simulink model "vehicles"  (R2020a)
settings: Solver=VariableStepAuto  StartTime=0.0  StopTime=10.0  RelTol=1e-3
undefined symbols (not defined in the file or in its folder): L, ld, psi_o1, psi_o10, psi_o2, psi_o3, psi_o4, psi_o5, psi_o6, psi_o7, psi_o8, psi_o9, X_last1, X_last10, X_last2, X_last3, X_last4, X_last5, X_last6, X_last7, X_last8, X_last9, X_o, X_o1, X_o10, X_o2, X_o3, X_o4, X_o5, X_o6, X_o7, X_o8, X_o9, xRef1, xRef10, xRef2, xRef3, xRef4, xRef5, xRef6, xRef7, xRef8, xRef9, Y_last1, Y_last10, Y_last2, Y_last3, Y_last4, Y_last5, Y_last6, Y_last7, Y_last8, Y_last9, Y_o, Y_o1, Y_o10, Y_o2, Y_o3, Y_o4, Y_o5 ... (+14)
libraries: autolibutils x40, autolibshared x30, robotalgslib x10, simulink x10, vdynlib x10
(part 1 of 18)
settings Model: Creator=Eskola  LastModifiedBy=Eskola

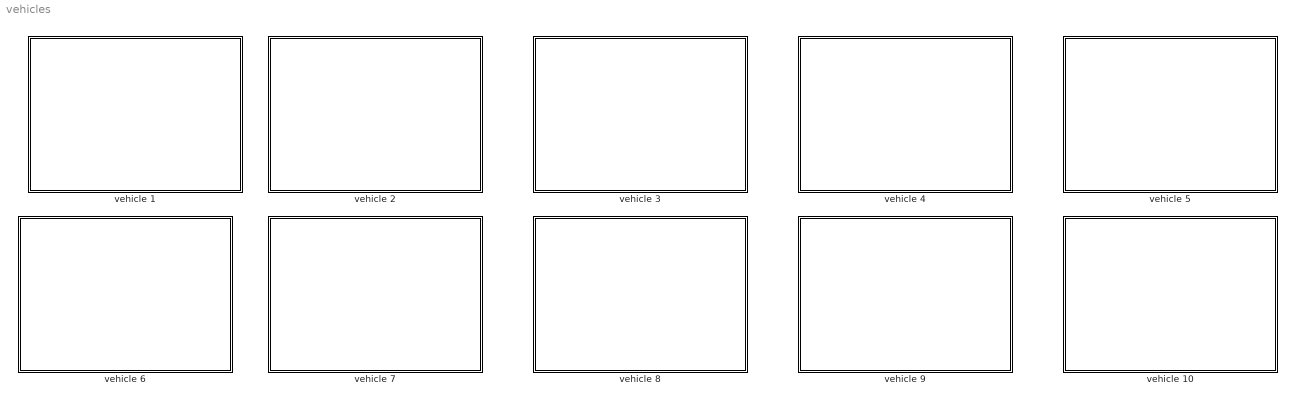
== system vehicles ==
  vehicle 1 : Subsystem
  vehicle 10 : Subsystem
  vehicle 2 : Subsystem
  vehicle 3 : Subsystem
  vehicle 4 : Subsystem
  vehicle 5 : Subsystem
  vehicle 6 : Subsystem
  vehicle 7 : Subsystem
  vehicle 8 : Subsystem
  vehicle 9 : Subsystem

== system vehicles/vehicle 1 ==
  note: Controller
  note: Vehicle Model
  note: Reference
  Bus to Mux1 : Subsystem
  Concatenate1 : Subsystem
  Constant3 : Constant  Value=X_o1
  Constant4 : Constant  Value=Y_o1
  Constant5 : Constant  Value=psi_o1
  Grade1 : Constant  Value=0
  Lateral and Longitudinal Controller1 : Subsystem
  Memory1 : Memory
  Powertrain & Driveline1 : Subsystem
      mask Display: image('vdbslibpt.png');
  Rate Transition1 : Subsystem
  Scope8 : Scope
  Simulation 3D Vehicle with Ground Following1 : vdynlib/Vehicle Scenarios/Sim3D/Sim3D Vehicle/Components/Simulation 3D Vehicle with Ground Following  Priority=-1  PassVehMesh=Small pickup truck  VehColor=Orange  InitialPos=[0,0,0]  InitialRot=[0, 0, 0]  ActorName=SimulinkVehicle1  SampleTime=-1  ActorType=SimulinkVehicle  ID=1  aMode=2  ActorTag=SimulinkVehicle1  CoordinateScheme=SAE
      settings: SourceProductBaseCode=VE
  Terminator{1..3,5..6} (5 alike) : Terminator
  Vehicle Body 3DOF Dual Track1 : autolibshared/Vehicle Body 3DOF Single Track  trackMode=Dual  inputMode=External longitudinal forces  frontSteerMode=on  rearSteerMode=off  windMode=off  muMode=off  extFMode=off  extMMode=off  extXo=on  extpsio=on  extxdoto=off  extro=off  extYo=on  extTamb=off  extydoto=off  aMode=2  NF=2  NR=2  m=2000  a=1.4  b=1.6  h=0.35  X_o=0  xdot_o=0  CalphaMode=off  sigmaMode=on  d=0  w=[1.4,1.4]  Cy_f=12e3  Cy_r=11e3  sigma_f=.1  sigma_r=.1  alpha_f_brk=[-.1 .1]  Cy_f_data=[-9e3 9e3]  alpha_r_brk=[-.1 .1]  Cy_r_data=[-9e3 9e3]  Y_o=0  ydot_o=0  Izz=4000  psi_o=0  r_o=0  Af=2  Cd=.3  Cl=.1  Cpm=.1  beta_w=[0:0.01:0.3]  Cs=[0:0.03:0.9]  Cym=[0:0.01:0.3]  Pabs=101325  Tair=273  g=9.81  mu=1  xdot_tol=.01  Fznom=5000  Fxtire_sat=7e4  Fytire_sat=7e4  longOff=0  latOff=0  vertOff=0  wrapAng=off
      settings: SourceProductBaseCode=PW,MT,VE,VP
  VelRefController1 : Subsystem
  Waypoints1 : Subsystem
  wires:
  Vehicle Body 3DOF Dual Track1/1 -> Rate Transition1/1(Info), Powertrain & Driveline1/3(VehFdbk), Bus to Mux1/1(Info)
  Concatenate1/1(AnF) -> Vehicle Body 3DOF Dual Track1/1
  Bus to Mux1/1(Pose) -> Lateral and Longitudinal Controller1/3(Pose)
  Memory1/1 -> VelRefController1/1(angVel)
  Lateral and Longitudinal Controller1/2(WheelSteeringAngle) -> Concatenate1/1(delta)
  Rate Transition1/3(Yaw) -> Simulation 3D Vehicle with Ground Following1/3
  Lateral and Longitudinal Controller1/4(DecelCmd) -> Powertrain & Driveline1/2(Decel)
  Rate Transition1/2(Y) -> Simulation 3D Vehicle with Ground Following1/2
  Lateral and Longitudinal Controller1/1(angVel) -> Memory1/1
  Bus to Mux1/2(x) -> Lateral and Longitudinal Controller1/6(xCar)
  Lateral and Longitudinal Controller1/3(AcelCmd) -> Powertrain & Driveline1/1(Acc)
  VelRefController1/1(VelRef) -> Lateral and Longitudinal Controller1/4(VelRef)
  Vehicle Body 3DOF Dual Track1/7 -> Terminator6/1
  Vehicle Body 3DOF Dual Track1/3 -> Terminator2/1
  Bus to Mux1/3(y) -> Lateral and Longitudinal Controller1/7(yCar)
  Constant5/1 -> Vehicle Body 3DOF Dual Track1/6
  Vehicle Body 3DOF Dual Track1/6 -> Terminator5/1
  Rate Transition1/1(X) -> Simulation 3D Vehicle with Ground Following1/1
  Powertrain & Driveline1/2(Rear Force) -> Vehicle Body 3DOF Dual Track1/3
  Vehicle Body 3DOF Dual Track1/4 -> Terminator1/1
  Constant3/1 -> Vehicle Body 3DOF Dual Track1/4
  Vehicle Body 3DOF Dual Track1/2 -> Lateral and Longitudinal Controller1/5(VelFdbk), Scope8/1
  Powertrain & Driveline1/1(Front Force) -> Vehicle Body 3DOF Dual Track1/2
  Vehicle Body 3DOF Dual Track1/5 -> Terminator3/1
  Waypoints1/1(WayPoints) -> Lateral and Longitudinal Controller1/1(Waypoints)
  Constant4/1 -> Vehicle Body 3DOF Dual Track1/5
  Grade1/1 -> Lateral and Longitudinal Controller1/2(Grade)

== system vehicles/vehicle 10 ==
  note: Reference
  note: Vehicle Model
  note: Controller
  Bus to Mux1 : Subsystem
  Concatenate1 : Subsystem
  Constant3 : Constant  Value=X_o10
  Constant4 : Constant  Value=Y_o10
  Constant5 : Constant  Value=psi_o10
  Grade1 : Constant  Value=0
  Lateral and Longitudinal Controller1 : Subsystem
  Memory1 : Memory
  Powertrain & Driveline1 : Subsystem
      mask Display: image('vdbslibpt.png');
  Rate Transition1 : Subsystem
  Scope8 : Scope
  Simulation 3D Vehicle with Ground Following1 : vdynlib/Vehicle Scenarios/Sim3D/Sim3D Vehicle/Components/Simulation 3D Vehicle with Ground Following  Priority=-1  PassVehMesh=Box truck  VehColor=Green  InitialPos=[0,0,0]  InitialRot=[0, 0, 0]  ActorName=SimulinkVehicle1  SampleTime=-1  ActorType=SimulinkVehicle  ID=1  aMode=2  ActorTag=SimulinkVehicle1  CoordinateScheme=SAE
      settings: SourceProductBaseCode=VE
  Terminator{1..3,5..6} (5 alike) : Terminator
  Vehicle Body 3DOF Dual Track1 : autolibshared/Vehicle Body 3DOF Single Track  trackMode=Dual  inputMode=External longitudinal forces  frontSteerMode=on  rearSteerMode=off  windMode=off  muMode=off  extFMode=off  extMMode=off  extXo=on  extpsio=on  extxdoto=off  extro=off  extYo=on  extTamb=off  extydoto=off  aMode=2  NF=2  NR=2  m=2000  a=1.4  b=1.6  h=0.35  X_o=0  xdot_o=0  CalphaMode=off  sigmaMode=on  d=0  w=[1.4,1.4]  Cy_f=12e3  Cy_r=11e3  sigma_f=.1  sigma_r=.1  alpha_f_brk=[-.1 .1]  Cy_f_data=[-9e3 9e3]  alpha_r_brk=[-.1 .1]  Cy_r_data=[-9e3 9e3]  Y_o=0  ydot_o=0  Izz=4000  psi_o=0  r_o=0  Af=2  Cd=.3  Cl=.1  Cpm=.1  beta_w=[0:0.01:0.3]  Cs=[0:0.03:0.9]  Cym=[0:0.01:0.3]  Pabs=101325  Tair=273  g=9.81  mu=1  xdot_tol=.01  Fznom=5000  Fxtire_sat=7e4  Fytire_sat=7e4  longOff=0  latOff=0  vertOff=0  wrapAng=off
      settings: SourceProductBaseCode=PW,MT,VE,VP
  VelRefController1 : Subsystem
  Waypoints1 : Subsystem
  wires:
  Grade1/1 -> Lateral and Longitudinal Controller1/2(Grade)
  Constant4/1 -> Vehicle Body 3DOF Dual Track1/5
  Waypoints1/1(WayPoints) -> Lateral and Longitudinal Controller1/1(Waypoints)
  Vehicle Body 3DOF Dual Track1/5 -> Terminator3/1
  Powertrain & Driveline1/1(Front Force) -> Vehicle Body 3DOF Dual Track1/2
  Vehicle Body 3DOF Dual Track1/2 -> Scope8/1, Lateral and Longitudinal Controller1/5(VelFdbk)
  Constant3/1 -> Vehicle Body 3DOF Dual Track1/4
  Vehicle Body 3DOF Dual Track1/4 -> Terminator1/1
  Powertrain & Driveline1/2(Rear Force) -> Vehicle Body 3DOF Dual Track1/3
  Rate Transition1/1(X) -> Simulation 3D Vehicle with Ground Following1/1
  Vehicle Body 3DOF Dual Track1/6 -> Terminator5/1
  Constant5/1 -> Vehicle Body 3DOF Dual Track1/6
  Bus to Mux1/3(y) -> Lateral and Longitudinal Controller1/7(yCar)
  Vehicle Body 3DOF Dual Track1/3 -> Terminator2/1
  Vehicle Body 3DOF Dual Track1/7 -> Terminator6/1
  VelRefController1/1(VelRef) -> Lateral and Longitudinal Controller1/4(VelRef)
  Lateral and Longitudinal Controller1/3(AcelCmd) -> Powertrain & Driveline1/1(Acc)
  Bus to Mux1/2(x) -> Lateral and Longitudinal Controller1/6(xCar)
  Lateral and Longitudinal Controller1/1(angVel) -> Memory1/1
  Rate Transition1/2(Y) -> Simulation 3D Vehicle with Ground Following1/2
  Lateral and Longitudinal Controller1/4(DecelCmd) -> Powertrain & Driveline1/2(Decel)
  Rate Transition1/3(Yaw) -> Simulation 3D Vehicle with Ground Following1/3
  Lateral and Longitudinal Controller1/2(WheelSteeringAngle) -> Concatenate1/1(delta)
  Memory1/1 -> VelRefController1/1(angVel)
  Bus to Mux1/1(Pose) -> Lateral and Longitudinal Controller1/3(Pose)
  Concatenate1/1(AnF) -> Vehicle Body 3DOF Dual Track1/1
  Vehicle Body 3DOF Dual Track1/1 -> Bus to Mux1/1(Info), Powertrain & Driveline1/3(VehFdbk), Rate Transition1/1(Info)

== system vehicles/vehicle 2 ==
  note: Reference
  note: Vehicle Model
  note: Controller
  Bus to Mux1 : Subsystem
  Concatenate1 : Subsystem
  Constant3 : Constant  Value=X_o2
  Constant4 : Constant  Value=Y_o2
  Constant5 : Constant  Value=psi_o2
  Grade1 : Constant  Value=0
  Lateral and Longitudinal Controller1 : Subsystem
  Memory1 : Memory
  Powertrain & Driveline1 : Subsystem
      mask Display: image('vdbslibpt.png');
  Rate Transition1 : Subsystem
  Scope8 : Scope
  Simulation 3D Vehicle with Ground Following1 : vdynlib/Vehicle Scenarios/Sim3D/Sim3D Vehicle/Components/Simulation 3D Vehicle with Ground Following  Priority=-1  PassVehMesh=Muscle car  VehColor=Blue  InitialPos=[0,0,0]  InitialRot=[0, 0, 0]  ActorName=SimulinkVehicle1  SampleTime=-1  ActorType=SimulinkVehicle  ID=1  aMode=2  ActorTag=SimulinkVehicle1  CoordinateScheme=SAE
      settings: SourceProductBaseCode=VE
  Terminator{1..3,5..6} (5 alike) : Terminator
  Vehicle Body 3DOF Dual Track1 : autolibshared/Vehicle Body 3DOF Single Track  trackMode=Dual  inputMode=External longitudinal forces  frontSteerMode=on  rearSteerMode=off  windMode=off  muMode=off  extFMode=off  extMMode=off  extXo=on  extpsio=on  extxdoto=off  extro=off  extYo=on  extTamb=off  extydoto=off  aMode=2  NF=2  NR=2  m=2000  a=1.4  b=1.6  h=0.35  X_o=0  xdot_o=0  CalphaMode=off  sigmaMode=on  d=0  w=[1.4,1.4]  Cy_f=12e3  Cy_r=11e3  sigma_f=.1  sigma_r=.1  alpha_f_brk=[-.1 .1]  Cy_f_data=[-9e3 9e3]  alpha_r_brk=[-.1 .1]  Cy_r_data=[-9e3 9e3]  Y_o=0  ydot_o=0  Izz=4000  psi_o=0  r_o=0  Af=2  Cd=.3  Cl=.1  Cpm=.1  beta_w=[0:0.01:0.3]  Cs=[0:0.03:0.9]  Cym=[0:0.01:0.3]  Pabs=101325  Tair=273  g=9.81  mu=1  xdot_tol=.01  Fznom=5000  Fxtire_sat=7e4  Fytire_sat=7e4  longOff=0  latOff=0  vertOff=0  wrapAng=off
      settings: SourceProductBaseCode=PW,MT,VE,VP
  VelRefController1 : Subsystem
  Waypoints1 : Subsystem
  wires:
  Grade1/1 -> Lateral and Longitudinal Controller1/2(Grade)
  Constant4/1 -> Vehicle Body 3DOF Dual Track1/5
  Waypoints1/1(WayPoints) -> Lateral and Longitudinal Controller1/1(Waypoints)
  Vehicle Body 3DOF Dual Track1/5 -> Terminator3/1
  Powertrain & Driveline1/1(Front Force) -> Vehicle Body 3DOF Dual Track1/2
  Vehicle Body 3DOF Dual Track1/2 -> Scope8/1, Lateral and Longitudinal Controller1/5(VelFdbk)
  Constant3/1 -> Vehicle Body 3DOF Dual Track1/4
  Vehicle Body 3DOF Dual Track1/4 -> Terminator1/1
  Powertrain & Driveline1/2(Rear Force) -> Vehicle Body 3DOF Dual Track1/3
  Rate Transition1/1(X) -> Simulation 3D Vehicle with Ground Following1/1
  Vehicle Body 3DOF Dual Track1/6 -> Terminator5/1
  Constant5/1 -> Vehicle Body 3DOF Dual Track1/6
  Bus to Mux1/3(y) -> Lateral and Longitudinal Controller1/7(yCar)
  Vehicle Body 3DOF Dual Track1/3 -> Terminator2/1
  Vehicle Body 3DOF Dual Track1/7 -> Terminator6/1
  VelRefController1/1(VelRef) -> Lateral and Longitudinal Controller1/4(VelRef)
  Lateral and Longitudinal Controller1/3(AcelCmd) -> Powertrain & Driveline1/1(Acc)
  Bus to Mux1/2(x) -> Lateral and Longitudinal Controller1/6(xCar)
  Lateral and Longitudinal Controller1/1(angVel) -> Memory1/1
  Rate Transition1/2(Y) -> Simulation 3D Vehicle with Ground Following1/2
  Lateral and Longitudinal Controller1/4(DecelCmd) -> Powertrain & Driveline1/2(Decel)
  Rate Transition1/3(Yaw) -> Simulation 3D Vehicle with Ground Following1/3
  Lateral and Longitudinal Controller1/2(WheelSteeringAngle) -> Concatenate1/1(delta)
  Memory1/1 -> VelRefController1/1(angVel)
  Bus to Mux1/1(Pose) -> Lateral and Longitudinal Controller1/3(Pose)
  Concatenate1/1(AnF) -> Vehicle Body 3DOF Dual Track1/1
  Vehicle Body 3DOF Dual Track1/1 -> Bus to Mux1/1(Info), Powertrain & Driveline1/3(VehFdbk), Rate Transition1/1(Info)

== system vehicles/vehicle 3 ==
  note: Controller
  note: Vehicle Model
  note: Reference
  Bus to Mux1 : Subsystem
  Concatenate1 : Subsystem
  Constant3 : Constant  Value=X_o3
  Constant4 : Constant  Value=Y_o3
  Constant5 : Constant  Value=psi_o3
  Grade1 : Constant  Value=0
  Lateral and Longitudinal Controller1 : Subsystem
  Memory1 : Memory
  Powertrain & Driveline1 : Subsystem
      mask Display: image('vdbslibpt.png');
  Rate Transition1 : Subsystem
  Scope8 : Scope
  Simulation 3D Vehicle with Ground Following1 : vdynlib/Vehicle Scenarios/Sim3D/Sim3D Vehicle/Components/Simulation 3D Vehicle with Ground Following  Priority=-1  PassVehMesh=Sedan  VehColor=Black  InitialPos=[0,0,0]  InitialRot=[0, 0, 0]  ActorName=SimulinkVehicle1  SampleTime=-1  ActorType=SimulinkVehicle  ID=1  aMode=2  ActorTag=SimulinkVehicle1  CoordinateScheme=SAE
      settings: SourceProductBaseCode=VE
  Terminator{1..3,5..6} (5 alike) : Terminator
  Vehicle Body 3DOF Dual Track1 : autolibshared/Vehicle Body 3DOF Single Track  trackMode=Dual  inputMode=External longitudinal forces  frontSteerMode=on  rearSteerMode=off  windMode=off  muMode=off  extFMode=off  extMMode=off  extXo=on  extpsio=on  extxdoto=off  extro=off  extYo=on  extTamb=off  extydoto=off  aMode=2  NF=2  NR=2  m=2000  a=1.4  b=1.6  h=0.35  X_o=0  xdot_o=0  CalphaMode=off  sigmaMode=on  d=0  w=[1.4,1.4]  Cy_f=12e3  Cy_r=11e3  sigma_f=.1  sigma_r=.1  alpha_f_brk=[-.1 .1]  Cy_f_data=[-9e3 9e3]  alpha_r_brk=[-.1 .1]  Cy_r_data=[-9e3 9e3]  Y_o=0  ydot_o=0  Izz=4000  psi_o=0  r_o=0  Af=2  Cd=.3  Cl=.1  Cpm=.1  beta_w=[0:0.01:0.3]  Cs=[0:0.03:0.9]  Cym=[0:0.01:0.3]  Pabs=101325  Tair=273  g=9.81  mu=1  xdot_tol=.01  Fznom=5000  Fxtire_sat=7e4  Fytire_sat=7e4  longOff=0  latOff=0  vertOff=0  wrapAng=off
      settings: SourceProductBaseCode=PW,MT,VE,VP
  VelRefController1 : Subsystem
  Waypoints1 : Subsystem
  wires:
  Vehicle Body 3DOF Dual Track1/1 -> Rate Transition1/1(Info), Powertrain & Driveline1/3(VehFdbk), Bus to Mux1/1(Info)
  Concatenate1/1(AnF) -> Vehicle Body 3DOF Dual Track1/1
  Bus to Mux1/1(Pose) -> Lateral and Longitudinal Controller1/3(Pose)
  Memory1/1 -> VelRefController1/1(angVel)
  Lateral and Longitudinal Controller1/2(WheelSteeringAngle) -> Concatenate1/1(delta)
  Rate Transition1/3(Yaw) -> Simulation 3D Vehicle with Ground Following1/3
  Lateral and Longitudinal Controller1/4(DecelCmd) -> Powertrain & Driveline1/2(Decel)
  Rate Transition1/2(Y) -> Simulation 3D Vehicle with Ground Following1/2
  Lateral and Longitudinal Controller1/1(angVel) -> Memory1/1
  Bus to Mux1/2(x) -> Lateral and Longitudinal Controller1/6(xCar)
  Lateral and Longitudinal Controller1/3(AcelCmd) -> Powertrain & Driveline1/1(Acc)
  VelRefController1/1(VelRef) -> Lateral and Longitudinal Controller1/4(VelRef)
  Vehicle Body 3DOF Dual Track1/7 -> Terminator6/1
  Vehicle Body 3DOF Dual Track1/3 -> Terminator2/1
  Bus to Mux1/3(y) -> Lateral and Longitudinal Controller1/7(yCar)
  Constant5/1 -> Vehicle Body 3DOF Dual Track1/6
  Vehicle Body 3DOF Dual Track1/6 -> Terminator5/1
  Rate Transition1/1(X) -> Simulation 3D Vehicle with Ground Following1/1
  Powertrain & Driveline1/2(Rear Force) -> Vehicle Body 3DOF Dual Track1/3
  Vehicle Body 3DOF Dual Track1/4 -> Terminator1/1
  Constant3/1 -> Vehicle Body 3DOF Dual Track1/4
  Vehicle Body 3DOF Dual Track1/2 -> Lateral and Longitudinal Controller1/5(VelFdbk), Scope8/1
  Powertrain & Driveline1/1(Front Force) -> Vehicle Body 3DOF Dual Track1/2
  Vehicle Body 3DOF Dual Track1/5 -> Terminator3/1
  Waypoints1/1(WayPoints) -> Lateral and Longitudinal Controller1/1(Waypoints)
  Constant4/1 -> Vehicle Body 3DOF Dual Track1/5
  Grade1/1 -> Lateral and Longitudinal Controller1/2(Grade)

== system vehicles/vehicle 4 ==
  note: Reference
  note: Vehicle Model
  note: Controller
  Bus to Mux1 : Subsystem
  Concatenate1 : Subsystem
  Constant3 : Constant  Value=X_o4
  Constant4 : Constant  Value=Y_o4
  Constant5 : Constant  Value=psi_o4
  Grade1 : Constant  Value=0
  Lateral and Longitudinal Controller1 : Subsystem
  Memory1 : Memory
  Powertrain & Driveline1 : Subsystem
      mask Display: image('vdbslibpt.png');
  Rate Transition1 : Subsystem
  Scope8 : Scope
  Simulation 3D Vehicle with Ground Following1 : vdynlib/Vehicle Scenarios/Sim3D/Sim3D Vehicle/Components/Simulation 3D Vehicle with Ground Following  Priority=-1  PassVehMesh=Sport utility vehicle  VehColor=Silver  InitialPos=[0,0,0]  InitialRot=[0, 0, 0]  ActorName=SimulinkVehicle2  SampleTime=-1  ActorType=SimulinkVehicle  ID=2  aMode=2  ActorTag=SimulinkVehicle2  CoordinateScheme=SAE
      settings: SourceProductBaseCode=VE
  Terminator{1..3,5..6} (5 alike) : Terminator
  Vehicle Body 3DOF Dual Track1 : autolibshared/Vehicle Body 3DOF Single Track  trackMode=Dual  inputMode=External longitudinal forces  frontSteerMode=on  rearSteerMode=off  windMode=off  muMode=off  extFMode=off  extMMode=off  extXo=on  extpsio=on  extxdoto=off  extro=off  extYo=on  extTamb=off  extydoto=off  aMode=2  NF=2  NR=2  m=2000  a=1.4  b=1.6  h=0.35  X_o=0  xdot_o=0  CalphaMode=off  sigmaMode=on  d=0  w=[1.4,1.4]  Cy_f=12e3  Cy_r=11e3  sigma_f=.1  sigma_r=.1  alpha_f_brk=[-.1 .1]  Cy_f_data=[-9e3 9e3]  alpha_r_brk=[-.1 .1]  Cy_r_data=[-9e3 9e3]  Y_o=0  ydot_o=0  Izz=4000  psi_o=0  r_o=0  Af=2  Cd=.3  Cl=.1  Cpm=.1  beta_w=[0:0.01:0.3]  Cs=[0:0.03:0.9]  Cym=[0:0.01:0.3]  Pabs=101325  Tair=273  g=9.81  mu=1  xdot_tol=.01  Fznom=5000  Fxtire_sat=7e4  Fytire_sat=7e4  longOff=0  latOff=0  vertOff=0  wrapAng=off
      settings: SourceProductBaseCode=PW,MT,VE,VP
  VelRefController1 : Subsystem
  Waypoints1 : Subsystem
  wires:
  Grade1/1 -> Lateral and Longitudinal Controller1/2(Grade)
  Constant4/1 -> Vehicle Body 3DOF Dual Track1/5
  Waypoints1/1(WayPoints) -> Lateral and Longitudinal Controller1/1(Waypoints)
  Vehicle Body 3DOF Dual Track1/5 -> Terminator3/1
  Powertrain & Driveline1/1(Front Force) -> Vehicle Body 3DOF Dual Track1/2
  Vehicle Body 3DOF Dual Track1/2 -> Scope8/1, Lateral and Longitudinal Controller1/5(VelFdbk)
  Constant3/1 -> Vehicle Body 3DOF Dual Track1/4
  Vehicle Body 3DOF Dual Track1/4 -> Terminator1/1
  Powertrain & Driveline1/2(Rear Force) -> Vehicle Body 3DOF Dual Track1/3
  Rate Transition1/1(X) -> Simulation 3D Vehicle with Ground Following1/1
  Vehicle Body 3DOF Dual Track1/6 -> Terminator5/1
  Constant5/1 -> Vehicle Body 3DOF Dual Track1/6
  Bus to Mux1/3(y) -> Lateral and Longitudinal Controller1/7(yCar)
  Vehicle Body 3DOF Dual Track1/3 -> Terminator2/1
  Vehicle Body 3DOF Dual Track1/7 -> Terminator6/1
  VelRefController1/1(VelRef) -> Lateral and Longitudinal Controller1/4(VelRef)
  Lateral and Longitudinal Controller1/3(AcelCmd) -> Powertrain & Driveline1/1(Acc)
  Bus to Mux1/2(x) -> Lateral and Longitudinal Controller1/6(xCar)
  Lateral and Longitudinal Controller1/1(angVel) -> Memory1/1
  Rate Transition1/2(Y) -> Simulation 3D Vehicle with Ground Following1/2
  Lateral and Longitudinal Controller1/4(DecelCmd) -> Powertrain & Driveline1/2(Decel)
  Rate Transition1/3(Yaw) -> Simulation 3D Vehicle with Ground Following1/3
  Lateral and Longitudinal Controller1/2(WheelSteeringAngle) -> Concatenate1/1(delta)
  Memory1/1 -> VelRefController1/1(angVel)
  Bus to Mux1/1(Pose) -> Lateral and Longitudinal Controller1/3(Pose)
  Concatenate1/1(AnF) -> Vehicle Body 3DOF Dual Track1/1
  Vehicle Body 3DOF Dual Track1/1 -> Bus to Mux1/1(Info), Powertrain & Driveline1/3(VehFdbk), Rate Transition1/1(Info)

== system vehicles/vehicle 5 ==
  note: Controller
  note: Vehicle Model
  note: Reference
  Bus to Mux1 : Subsystem
  Concatenate1 : Subsystem
  Constant3 : Constant  Value=X_o5
  Constant4 : Constant  Value=Y_o5
  Constant5 : Constant  Value=psi_o5
  Grade1 : Constant  Value=0
  Lateral and Longitudinal Controller1 : Subsystem
  Memory1 : Memory
  Powertrain & Driveline1 : Subsystem
      mask Display: image('vdbslibpt.png');
  Rate Transition1 : Subsystem
  Scope8 : Scope
  Simulation 3D Vehicle with Ground Following1 : vdynlib/Vehicle Scenarios/Sim3D/Sim3D Vehicle/Components/Simulation 3D Vehicle with Ground Following  Priority=-1  PassVehMesh=Hatchback  VehColor=Red  InitialPos=[0,0,0]  InitialRot=[0, 0, 0]  ActorName=SimulinkVehicle3  SampleTime=-1  ActorType=SimulinkVehicle  ID=3  aMode=2  ActorTag=SimulinkVehicle3  CoordinateScheme=SAE
      settings: SourceProductBaseCode=VE
  Terminator{1..3,5..6} (5 alike) : Terminator
  Vehicle Body 3DOF Dual Track1 : autolibshared/Vehicle Body 3DOF Single Track  trackMode=Dual  inputMode=External longitudinal forces  frontSteerMode=on  rearSteerMode=off  windMode=off  muMode=off  extFMode=off  extMMode=off  extXo=on  extpsio=on  extxdoto=off  extro=off  extYo=on  extTamb=off  extydoto=off  aMode=2  NF=2  NR=2  m=2000  a=1.4  b=1.6  h=0.35  X_o=0  xdot_o=0  CalphaMode=off  sigmaMode=on  d=0  w=[1.4,1.4]  Cy_f=12e3  Cy_r=11e3  sigma_f=.1  sigma_r=.1  alpha_f_brk=[-.1 .1]  Cy_f_data=[-9e3 9e3]  alpha_r_brk=[-.1 .1]  Cy_r_data=[-9e3 9e3]  Y_o=0  ydot_o=0  Izz=4000  psi_o=0  r_o=0  Af=2  Cd=.3  Cl=.1  Cpm=.1  beta_w=[0:0.01:0.3]  Cs=[0:0.03:0.9]  Cym=[0:0.01:0.3]  Pabs=101325  Tair=273  g=9.81  mu=1  xdot_tol=.01  Fznom=5000  Fxtire_sat=7e4  Fytire_sat=7e4  longOff=0  latOff=0  vertOff=0  wrapAng=off
      settings: SourceProductBaseCode=PW,MT,VE,VP
  VelRefController1 : Subsystem
  Waypoints1 : Subsystem
  wires:
  Vehicle Body 3DOF Dual Track1/1 -> Rate Transition1/1(Info), Powertrain & Driveline1/3(VehFdbk), Bus to Mux1/1(Info)
  Concatenate1/1(AnF) -> Vehicle Body 3DOF Dual Track1/1
  Bus to Mux1/1(Pose) -> Lateral and Longitudinal Controller1/3(Pose)
  Memory1/1 -> VelRefController1/1(angVel)
  Lateral and Longitudinal Controller1/2(WheelSteeringAngle) -> Concatenate1/1(delta)
  Rate Transition1/3(Yaw) -> Simulation 3D Vehicle with Ground Following1/3
  Lateral and Longitudinal Controller1/4(DecelCmd) -> Powertrain & Driveline1/2(Decel)
  Rate Transition1/2(Y) -> Simulation 3D Vehicle with Ground Following1/2
  Lateral and Longitudinal Controller1/1(angVel) -> Memory1/1
  Bus to Mux1/2(x) -> Lateral and Longitudinal Controller1/6(xCar)
  Lateral and Longitudinal Controller1/3(AcelCmd) -> Powertrain & Driveline1/1(Acc)
  VelRefController1/1(VelRef) -> Lateral and Longitudinal Controller1/4(VelRef)
  Vehicle Body 3DOF Dual Track1/7 -> Terminator6/1
  Vehicle Body 3DOF Dual Track1/3 -> Terminator2/1
  Bus to Mux1/3(y) -> Lateral and Longitudinal Controller1/7(yCar)
  Constant5/1 -> Vehicle Body 3DOF Dual Track1/6
  Vehicle Body 3DOF Dual Track1/6 -> Terminator5/1
  Rate Transition1/1(X) -> Simulation 3D Vehicle with Ground Following1/1
  Powertrain & Driveline1/2(Rear Force) -> Vehicle Body 3DOF Dual Track1/3
  Vehicle Body 3DOF Dual Track1/4 -> Terminator1/1
  Constant3/1 -> Vehicle Body 3DOF Dual Track1/4
  Vehicle Body 3DOF Dual Track1/2 -> Lateral and Longitudinal Controller1/5(VelFdbk), Scope8/1
  Powertrain & Driveline1/1(Front Force) -> Vehicle Body 3DOF Dual Track1/2
  Vehicle Body 3DOF Dual Track1/5 -> Terminator3/1
  Waypoints1/1(WayPoints) -> Lateral and Longitudinal Controller1/1(Waypoints)
  Constant4/1 -> Vehicle Body 3DOF Dual Track1/5
  Grade1/1 -> Lateral and Longitudinal Controller1/2(Grade)

== system vehicles/vehicle 6 ==
  note: Reference
  note: Vehicle Model
  note: Controller
  Bus to Mux1 : Subsystem
  Concatenate1 : Subsystem
  Constant3 : Constant  Value=X_o6
  Constant4 : Constant  Value=Y_o6
  Constant5 : Constant  Value=psi_o6
  Grade1 : Constant  Value=0
  Lateral and Longitudinal Controller1 : Subsystem
  Memory1 : Memory
  Powertrain & Driveline1 : Subsystem
      mask Display: image('vdbslibpt.png');
  Rate Transition1 : Subsystem
  Scope8 : Scope
  Simulation 3D Vehicle with Ground Following1 : vdynlib/Vehicle Scenarios/Sim3D/Sim3D Vehicle/Components/Simulation 3D Vehicle with Ground Following  Priority=-1  PassVehMesh=Box truck  VehColor=Green  InitialPos=[0,0,0]  InitialRot=[0, 0, 0]  ActorName=SimulinkVehicle2  SampleTime=-1  ActorType=SimulinkVehicle  ID=2  aMode=2  ActorTag=SimulinkVehicle2  CoordinateScheme=SAE
      settings: SourceProductBaseCode=VE
  Terminator{1..3,5..6} (5 alike) : Terminator
  Vehicle Body 3DOF Dual Track1 : autolibshared/Vehicle Body 3DOF Single Track  trackMode=Dual  inputMode=External longitudinal forces  frontSteerMode=on  rearSteerMode=off  windMode=off  muMode=off  extFMode=off  extMMode=off  extXo=on  extpsio=on  extxdoto=off  extro=off  extYo=on  extTamb=off  extydoto=off  aMode=2  NF=2  NR=2  m=2000  a=1.4  b=1.6  h=0.35  X_o=0  xdot_o=0  CalphaMode=off  sigmaMode=on  d=0  w=[1.4,1.4]  Cy_f=12e3  Cy_r=11e3  sigma_f=.1  sigma_r=.1  alpha_f_brk=[-.1 .1]  Cy_f_data=[-9e3 9e3]  alpha_r_brk=[-.1 .1]  Cy_r_data=[-9e3 9e3]  Y_o=0  ydot_o=0  Izz=4000  psi_o=0  r_o=0  Af=2  Cd=.3  Cl=.1  Cpm=.1  beta_w=[0:0.01:0.3]  Cs=[0:0.03:0.9]  Cym=[0:0.01:0.3]  Pabs=101325  Tair=273  g=9.81  mu=1  xdot_tol=.01  Fznom=5000  Fxtire_sat=7e4  Fytire_sat=7e4  longOff=0  latOff=0  vertOff=0  wrapAng=off
      settings: SourceProductBaseCode=PW,MT,VE,VP
  VelRefController1 : Subsystem
  Waypoints1 : Subsystem
  wires:
  Grade1/1 -> Lateral and Longitudinal Controller1/2(Grade)
  Constant4/1 -> Vehicle Body 3DOF Dual Track1/5
  Waypoints1/1(WayPoints) -> Lateral and Longitudinal Controller1/1(Waypoints)
  Vehicle Body 3DOF Dual Track1/5 -> Terminator3/1
  Powertrain & Driveline1/1(Front Force) -> Vehicle Body 3DOF Dual Track1/2
  Vehicle Body 3DOF Dual Track1/2 -> Scope8/1, Lateral and Longitudinal Controller1/5(VelFdbk)
  Constant3/1 -> Vehicle Body 3DOF Dual Track1/4
  Vehicle Body 3DOF Dual Track1/4 -> Terminator1/1
  Powertrain & Driveline1/2(Rear Force) -> Vehicle Body 3DOF Dual Track1/3
  Rate Transition1/1(X) -> Simulation 3D Vehicle with Ground Following1/1
  Vehicle Body 3DOF Dual Track1/6 -> Terminator5/1
  Constant5/1 -> Vehicle Body 3DOF Dual Track1/6
  Bus to Mux1/3(y) -> Lateral and Longitudinal Controller1/7(yCar)
  Vehicle Body 3DOF Dual Track1/3 -> Terminator2/1
  Vehicle Body 3DOF Dual Track1/7 -> Terminator6/1
  VelRefController1/1(VelRef) -> Lateral and Longitudinal Controller1/4(VelRef)
  Lateral and Longitudinal Controller1/3(AcelCmd) -> Powertrain & Driveline1/1(Acc)
  Bus to Mux1/2(x) -> Lateral and Longitudinal Controller1/6(xCar)
  Lateral and Longitudinal Controller1/1(angVel) -> Memory1/1
  Rate Transition1/2(Y) -> Simulation 3D Vehicle with Ground Following1/2
  Lateral and Longitudinal Controller1/4(DecelCmd) -> Powertrain & Driveline1/2(Decel)
  Rate Transition1/3(Yaw) -> Simulation 3D Vehicle with Ground Following1/3
  Lateral and Longitudinal Controller1/2(WheelSteeringAngle) -> Concatenate1/1(delta)
  Memory1/1 -> VelRefController1/1(angVel)
  Bus to Mux1/1(Pose) -> Lateral and Longitudinal Controller1/3(Pose)
  Concatenate1/1(AnF) -> Vehicle Body 3DOF Dual Track1/1
  Vehicle Body 3DOF Dual Track1/1 -> Bus to Mux1/1(Info), Powertrain & Driveline1/3(VehFdbk), Rate Transition1/1(Info)

== system vehicles/vehicle 7 ==
  note: Controller
  note: Vehicle Model
  note: Reference
  Bus to Mux1 : Subsystem
  Concatenate1 : Subsystem
  Constant3 : Constant  Value=X_o7
  Constant4 : Constant  Value=Y_o7
  Constant5 : Constant  Value=psi_o7
  Grade1 : Constant  Value=0
  Lateral and Longitudinal Controller1 : Subsystem
  Memory1 : Memory
  Powertrain & Driveline1 : Subsystem
      mask Display: image('vdbslibpt.png');
  Rate Transition1 : Subsystem
  Scope8 : Scope
  Simulation 3D Vehicle with Ground Following1 : vdynlib/Vehicle Scenarios/Sim3D/Sim3D Vehicle/Components/Simulation 3D Vehicle with Ground Following  Priority=-1  PassVehMesh=Box truck  VehColor=Green  InitialPos=[0,0,0]  InitialRot=[0, 0, 0]  ActorName=SimulinkVehicle3  SampleTime=-1  ActorType=SimulinkVehicle  ID=3  aMode=2  ActorTag=SimulinkVehicle3  CoordinateScheme=SAE
      settings: SourceProductBaseCode=VE
  Terminator{1..3,5..6} (5 alike) : Terminator
  Vehicle Body 3DOF Dual Track1 : autolibshared/Vehicle Body 3DOF Single Track  trackMode=Dual  inputMode=External longitudinal forces  frontSteerMode=on  rearSteerMode=off  windMode=off  muMode=off  extFMode=off  extMMode=off  extXo=on  extpsio=on  extxdoto=off  extro=off  extYo=on  extTamb=off  extydoto=off  aMode=2  NF=2  NR=2  m=2000  a=1.4  b=1.6  h=0.35  X_o=0  xdot_o=0  CalphaMode=off  sigmaMode=on  d=0  w=[1.4,1.4]  Cy_f=12e3  Cy_r=11e3  sigma_f=.1  sigma_r=.1  alpha_f_brk=[-.1 .1]  Cy_f_data=[-9e3 9e3]  alpha_r_brk=[-.1 .1]  Cy_r_data=[-9e3 9e3]  Y_o=0  ydot_o=0  Izz=4000  psi_o=0  r_o=0  Af=2  Cd=.3  Cl=.1  Cpm=.1  beta_w=[0:0.01:0.3]  Cs=[0:0.03:0.9]  Cym=[0:0.01:0.3]  Pabs=101325  Tair=273  g=9.81  mu=1  xdot_tol=.01  Fznom=5000  Fxtire_sat=7e4  Fytire_sat=7e4  longOff=0  latOff=0  vertOff=0  wrapAng=off
      settings: SourceProductBaseCode=PW,MT,VE,VP
  VelRefController1 : Subsystem
  Waypoints1 : Subsystem
  wires:
  Vehicle Body 3DOF Dual Track1/1 -> Rate Transition1/1(Info), Powertrain & Driveline1/3(VehFdbk), Bus to Mux1/1(Info)
  Concatenate1/1(AnF) -> Vehicle Body 3DOF Dual Track1/1
  Bus to Mux1/1(Pose) -> Lateral and Longitudinal Controller1/3(Pose)
  Memory1/1 -> VelRefController1/1(angVel)
  Lateral and Longitudinal Controller1/2(WheelSteeringAngle) -> Concatenate1/1(delta)
  Rate Transition1/3(Yaw) -> Simulation 3D Vehicle with Ground Following1/3
  Lateral and Longitudinal Controller1/4(DecelCmd) -> Powertrain & Driveline1/2(Decel)
  Rate Transition1/2(Y) -> Simulation 3D Vehicle with Ground Following1/2
  Lateral and Longitudinal Controller1/1(angVel) -> Memory1/1
  Bus to Mux1/2(x) -> Lateral and Longitudinal Controller1/6(xCar)
  Lateral and Longitudinal Controller1/3(AcelCmd) -> Powertrain & Driveline1/1(Acc)
  VelRefController1/1(VelRef) -> Lateral and Longitudinal Controller1/4(VelRef)
  Vehicle Body 3DOF Dual Track1/7 -> Terminator6/1
  Vehicle Body 3DOF Dual Track1/3 -> Terminator2/1
  Bus to Mux1/3(y) -> Lateral and Longitudinal Controller1/7(yCar)
  Constant5/1 -> Vehicle Body 3DOF Dual Track1/6
  Vehicle Body 3DOF Dual Track1/6 -> Terminator5/1
  Rate Transition1/1(X) -> Simulation 3D Vehicle with Ground Following1/1
  Powertrain & Driveline1/2(Rear Force) -> Vehicle Body 3DOF Dual Track1/3
  Vehicle Body 3DOF Dual Track1/4 -> Terminator1/1
  Constant3/1 -> Vehicle Body 3DOF Dual Track1/4
  Vehicle Body 3DOF Dual Track1/2 -> Lateral and Longitudinal Controller1/5(VelFdbk), Scope8/1
  Powertrain & Driveline1/1(Front Force) -> Vehicle Body 3DOF Dual Track1/2
  Vehicle Body 3DOF Dual Track1/5 -> Terminator3/1
  Waypoints1/1(WayPoints) -> Lateral and Longitudinal Controller1/1(Waypoints)
  Constant4/1 -> Vehicle Body 3DOF Dual Track1/5
  Grade1/1 -> Lateral and Longitudinal Controller1/2(Grade)

== system vehicles/vehicle 8 ==
  note: Reference
  note: Vehicle Model
  note: Controller
  Bus to Mux1 : Subsystem
  Concatenate1 : Subsystem
  Constant3 : Constant  Value=X_o8
  Constant4 : Constant  Value=Y_o8
  Constant5 : Constant  Value=psi_o8
  Grade1 : Constant  Value=0
  Lateral and Longitudinal Controller1 : Subsystem
  Memory1 : Memory
  Powertrain & Driveline1 : Subsystem
      mask Display: image('vdbslibpt.png');
  Rate Transition1 : Subsystem
  Scope8 : Scope
  Simulation 3D Vehicle with Ground Following1 : vdynlib/Vehicle Scenarios/Sim3D/Sim3D Vehicle/Components/Simulation 3D Vehicle with Ground Following  Priority=-1  PassVehMesh=Box truck  VehColor=Green  InitialPos=[0,0,0]  InitialRot=[0, 0, 0]  ActorName=SimulinkVehicle4  SampleTime=-1  ActorType=SimulinkVehicle  ID=4  aMode=2  ActorTag=SimulinkVehicle4  CoordinateScheme=SAE
      settings: SourceProductBaseCode=VE
  Terminator{1..3,5..6} (5 alike) : Terminator
  Vehicle Body 3DOF Dual Track1 : autolibshared/Vehicle Body 3DOF Single Track  trackMode=Dual  inputMode=External longitudinal forces  frontSteerMode=on  rearSteerMode=off  windMode=off  muMode=off  extFMode=off  extMMode=off  extXo=on  extpsio=on  extxdoto=off  extro=off  extYo=on  extTamb=off  extydoto=off  aMode=2  NF=2  NR=2  m=2000  a=1.4  b=1.6  h=0.35  X_o=0  xdot_o=0  CalphaMode=off  sigmaMode=on  d=0  w=[1.4,1.4]  Cy_f=12e3  Cy_r=11e3  sigma_f=.1  sigma_r=.1  alpha_f_brk=[-.1 .1]  Cy_f_data=[-9e3 9e3]  alpha_r_brk=[-.1 .1]  Cy_r_data=[-9e3 9e3]  Y_o=0  ydot_o=0  Izz=4000  psi_o=0  r_o=0  Af=2  Cd=.3  Cl=.1  Cpm=.1  beta_w=[0:0.01:0.3]  Cs=[0:0.03:0.9]  Cym=[0:0.01:0.3]  Pabs=101325  Tair=273  g=9.81  mu=1  xdot_tol=.01  Fznom=5000  Fxtire_sat=7e4  Fytire_sat=7e4  longOff=0  latOff=0  vertOff=0  wrapAng=off
      settings: SourceProductBaseCode=PW,MT,VE,VP
  VelRefController1 : Subsystem
  Waypoints1 : Subsystem
  wires:
  Grade1/1 -> Lateral and Longitudinal Controller1/2(Grade)
  Constant4/1 -> Vehicle Body 3DOF Dual Track1/5
  Waypoints1/1(WayPoints) -> Lateral and Longitudinal Controller1/1(Waypoints)
  Vehicle Body 3DOF Dual Track1/5 -> Terminator3/1
  Powertrain & Driveline1/1(Front Force) -> Vehicle Body 3DOF Dual Track1/2
  Vehicle Body 3DOF Dual Track1/2 -> Scope8/1, Lateral and Longitudinal Controller1/5(VelFdbk)
  Constant3/1 -> Vehicle Body 3DOF Dual Track1/4
  Vehicle Body 3DOF Dual Track1/4 -> Terminator1/1
  Powertrain & Driveline1/2(Rear Force) -> Vehicle Body 3DOF Dual Track1/3
  Rate Transition1/1(X) -> Simulation 3D Vehicle with Ground Following1/1
  Vehicle Body 3DOF Dual Track1/6 -> Terminator5/1
  Constant5/1 -> Vehicle Body 3DOF Dual Track1/6
  Bus to Mux1/3(y) -> Lateral and Longitudinal Controller1/7(yCar)
  Vehicle Body 3DOF Dual Track1/3 -> Terminator2/1
  Vehicle Body 3DOF Dual Track1/7 -> Terminator6/1
  VelRefController1/1(VelRef) -> Lateral and Longitudinal Controller1/4(VelRef)
  Lateral and Longitudinal Controller1/3(AcelCmd) -> Powertrain & Driveline1/1(Acc)
  Bus to Mux1/2(x) -> Lateral and Longitudinal Controller1/6(xCar)
  Lateral and Longitudinal Controller1/1(angVel) -> Memory1/1
  Rate Transition1/2(Y) -> Simulation 3D Vehicle with Ground Following1/2
  Lateral and Longitudinal Controller1/4(DecelCmd) -> Powertrain & Driveline1/2(Decel)
  Rate Transition1/3(Yaw) -> Simulation 3D Vehicle with Ground Following1/3
  Lateral and Longitudinal Controller1/2(WheelSteeringAngle) -> Concatenate1/1(delta)
  Memory1/1 -> VelRefController1/1(angVel)
  Bus to Mux1/1(Pose) -> Lateral and Longitudinal Controller1/3(Pose)
  Concatenate1/1(AnF) -> Vehicle Body 3DOF Dual Track1/1
  Vehicle Body 3DOF Dual Track1/1 -> Bus to Mux1/1(Info), Powertrain & Driveline1/3(VehFdbk), Rate Transition1/1(Info)

== system vehicles/vehicle 9 ==
  note: Controller
  note: Vehicle Model
  note: Reference
  Bus to Mux1 : Subsystem
  Concatenate1 : Subsystem
  Constant3 : Constant  Value=X_o9
  Constant4 : Constant  Value=Y_o9
  Constant5 : Constant  Value=psi_o9
  Grade1 : Constant  Value=0
  Lateral and Longitudinal Controller1 : Subsystem
  Memory1 : Memory
  Powertrain & Driveline1 : Subsystem
      mask Display: image('vdbslibpt.png');
  Rate Transition1 : Subsystem
  Scope8 : Scope
  Simulation 3D Vehicle with Ground Following1 : vdynlib/Vehicle Scenarios/Sim3D/Sim3D Vehicle/Components/Simulation 3D Vehicle with Ground Following  Priority=-1  PassVehMesh=Box truck  VehColor=Green  InitialPos=[0,0,0]  InitialRot=[0, 0, 0]  ActorName=SimulinkVehicle5  SampleTime=-1  ActorType=SimulinkVehicle  ID=5  aMode=2  ActorTag=SimulinkVehicle5  CoordinateScheme=SAE
      settings: SourceProductBaseCode=VE
  Terminator{1..3,5..6} (5 alike) : Terminator
  Vehicle Body 3DOF Dual Track1 : autolibshared/Vehicle Body 3DOF Single Track  trackMode=Dual  inputMode=External longitudinal forces  frontSteerMode=on  rearSteerMode=off  windMode=off  muMode=off  extFMode=off  extMMode=off  extXo=on  extpsio=on  extxdoto=off  extro=off  extYo=on  extTamb=off  extydoto=off  aMode=2  NF=2  NR=2  m=2000  a=1.4  b=1.6  h=0.35  X_o=0  xdot_o=0  CalphaMode=off  sigmaMode=on  d=0  w=[1.4,1.4]  Cy_f=12e3  Cy_r=11e3  sigma_f=.1  sigma_r=.1  alpha_f_brk=[-.1 .1]  Cy_f_data=[-9e3 9e3]  alpha_r_brk=[-.1 .1]  Cy_r_data=[-9e3 9e3]  Y_o=0  ydot_o=0  Izz=4000  psi_o=0  r_o=0  Af=2  Cd=.3  Cl=.1  Cpm=.1  beta_w=[0:0.01:0.3]  Cs=[0:0.03:0.9]  Cym=[0:0.01:0.3]  Pabs=101325  Tair=273  g=9.81  mu=1  xdot_tol=.01  Fznom=5000  Fxtire_sat=7e4  Fytire_sat=7e4  longOff=0  latOff=0  vertOff=0  wrapAng=off
      settings: SourceProductBaseCode=PW,MT,VE,VP
  VelRefController1 : Subsystem
  Waypoints1 : Subsystem
  wires:
  Vehicle Body 3DOF Dual Track1/1 -> Rate Transition1/1(Info), Powertrain & Driveline1/3(VehFdbk), Bus to Mux1/1(Info)
  Concatenate1/1(AnF) -> Vehicle Body 3DOF Dual Track1/1
  Bus to Mux1/1(Pose) -> Lateral and Longitudinal Controller1/3(Pose)
  Memory1/1 -> VelRefController1/1(angVel)
  Lateral and Longitudinal Controller1/2(WheelSteeringAngle) -> Concatenate1/1(delta)
  Rate Transition1/3(Yaw) -> Simulation 3D Vehicle with Ground Following1/3
  Lateral and Longitudinal Controller1/4(DecelCmd) -> Powertrain & Driveline1/2(Decel)
  Rate Transition1/2(Y) -> Simulation 3D Vehicle with Ground Following1/2
  Lateral and Longitudinal Controller1/1(angVel) -> Memory1/1
  Bus to Mux1/2(x) -> Lateral and Longitudinal Controller1/6(xCar)
  Lateral and Longitudinal Controller1/3(AcelCmd) -> Powertrain & Driveline1/1(Acc)
  VelRefController1/1(VelRef) -> Lateral and Longitudinal Controller1/4(VelRef)
  Vehicle Body 3DOF Dual Track1/7 -> Terminator6/1
  Vehicle Body 3DOF Dual Track1/3 -> Terminator2/1
  Bus to Mux1/3(y) -> Lateral and Longitudinal Controller1/7(yCar)
  Constant5/1 -> Vehicle Body 3DOF Dual Track1/6
  Vehicle Body 3DOF Dual Track1/6 -> Terminator5/1
  Rate Transition1/1(X) -> Simulation 3D Vehicle with Ground Following1/1
  Powertrain & Driveline1/2(Rear Force) -> Vehicle Body 3DOF Dual Track1/3
  Vehicle Body 3DOF Dual Track1/4 -> Terminator1/1
  Constant3/1 -> Vehicle Body 3DOF Dual Track1/4
  Vehicle Body 3DOF Dual Track1/2 -> Lateral and Longitudinal Controller1/5(VelFdbk), Scope8/1
  Powertrain & Driveline1/1(Front Force) -> Vehicle Body 3DOF Dual Track1/2
  Vehicle Body 3DOF Dual Track1/5 -> Terminator3/1
  Waypoints1/1(WayPoints) -> Lateral and Longitudinal Controller1/1(Waypoints)
  Constant4/1 -> Vehicle Body 3DOF Dual Track1/5
  Grade1/1 -> Lateral and Longitudinal Controller1/2(Grade)

== system vehicles/vehicle 1/Bus to Mux1 ==
  Info : Inport
  Bus Selector1 : BusSelector  OutputSignals=InertFrm.Cg.Disp.X,InertFrm.Cg.Disp.Y,InertFrm.Cg.Ang.psi
  Mux : Mux  Inputs=3
  Pose : Outport
  x : Outport  Port=2
  y : Outport  Port=3
  wires:
  Bus Selector1/3 -> Mux/3  "<psi>"
  Bus Selector1/1 -> Mux/1, x/1  "<X>"
  Mux/1 -> Pose/1
  Bus Selector1/2 -> y/1, Mux/2  "<Y>"
  Info/1 -> Bus Selector1/1

== system vehicles/vehicle 1/Concatenate1 ==
  delta : Inport
  Matrix Concatenate : Concatenate
  AnF : Outport  VectorParamsAs1DForOutWhenUnconnected=off
  wires:
  Matrix Concatenate/1 -> AnF/1
  delta/1 -> Matrix Concatenate/2, Matrix Concatenate/1

== system vehicles/vehicle 1/Lateral and Longitudinal Controller1 ==
  Waypoints : Inport
  Grade : Inport  Port=2
  Pose : Inport  Port=3
  VelRef : Inport  Port=4
  VelFdbk : Inport  Port=5
  xCar : Inport  Port=6
  yCar : Inport  Port=7
  Longitudinal Driver : autolibshared/Longitudinal Driver  extAccelOvr=off  extDecelOvr=off  extAccelHld=off  extDecelHld=off  extAccelZero=off  extDecelZero=off  cntrlType=PI  shftType=None  velUnits=m/s  gearOut=off  Kp=700  Ki=1  Kff=.1  Kg=0  VehVelVec=[0 100]  KffVec=[.1 .1]  KpVec=[10 10]  KiVec=[5 5]  KgVec=[0 0]  m=1500  Kpt=3000  tau=.1  L=2  aR=200  bR=2.5  cR=.5  g=9.81  vnom=9  Kaw=1  tauerr=.01  tauPt=2  GearInit=0  tShift=.1  pdlVec=[0.1 0.4 0.5 0.9]  upShftTbl=[-1 12.9375 26.4375 39.9375 51.18749999999999 62.4375 72.84375 83.25;-1 16.3125 29.8125 43.3125 54.5624 65.8125 76.78125 87.75;-1 19.6875 33.1875 46.68749999999999 57.9375 69.1875 80.71875 92.25;-1 33 52.5 77.25 100.5 138.75 161.875 185]  dwnShftTbl=[1 9.5625 23.0625 36.5625 47.8125 59.0625 68.90625 78.75;1 12.9375 26.4375 39.9375 51.18749999999999 62.4375 72.84375 83.25;1 16.3125 29.8125 43.3125 54.562499 65.8125 76.78125 87.75;1 19.6875 33.1875 46.68749999999999 57.9375 69.1875 80.71875 92.25]  tClutch=.5  tRev=.5  tPark=120  aMode=2  UpGearVec="[0  1  2  3  4  5  6  7]"  DownGearVec="[1  2  3  4  5  6  7  8]"
      settings: SourceProductBaseCode=PW,MT,VE,VP
  Pure Pursuit Controller : Subsystem
  Scope : Scope
  Scope1 : Scope
  Stop-system : Subsystem
  Terminator10 : Terminator
  angVel : Outport
  WheelSteeringAngle : Outport  Port=2
  AcelCmd : Outport  Port=3
  DecelCmd : Outport  Port=4
  wires:
  Pure Pursuit Controller/1(delta) -> WheelSteeringAngle/1
  Waypoints/1 -> Pure Pursuit Controller/2(Waypoints)
  Pose/1 -> Pure Pursuit Controller/1(Pose)
  Grade/1 -> Longitudinal Driver/3
  Longitudinal Driver/3 -> Stop-system/3(decel)
  VelRef/1 -> Longitudinal Driver/1
  VelFdbk/1 -> Longitudinal Driver/2
  Longitudinal Driver/2 -> Stop-system/1(acel)
  Longitudinal Driver/1 -> Terminator10/1
  Pure Pursuit Controller/2(AngularVelocity) -> angVel/1
  xCar/1 -> Stop-system/2(xCar)
  yCar/1 -> Stop-system/4(yCar)
  Stop-system/1(AcelCmd) -> Scope/1, AcelCmd/1
  Stop-system/2(DecelCmd) -> Scope1/1, DecelCmd/1

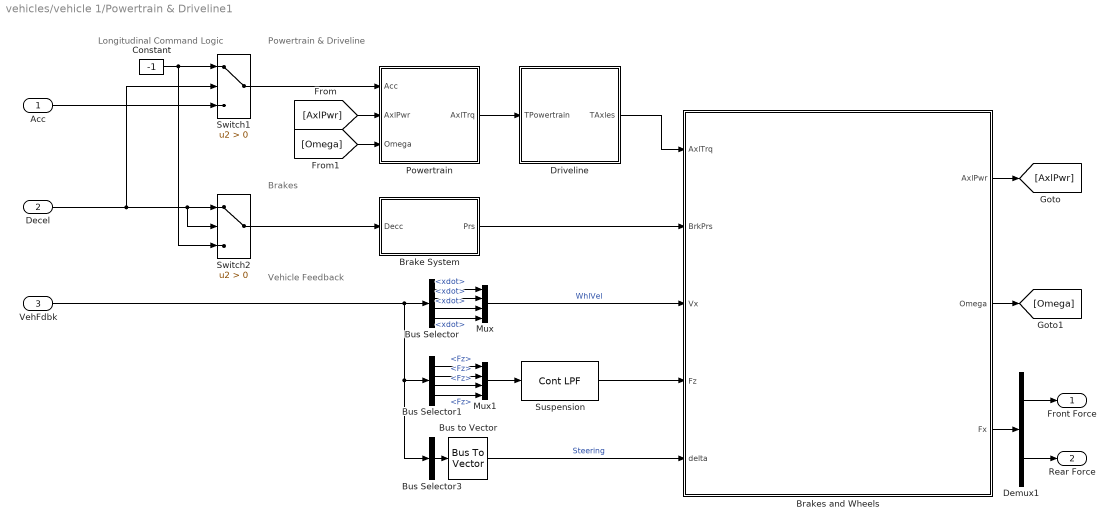
== system vehicles/vehicle 1/Powertrain & Driveline1 ==
  note: Vehicle Feedback
  note: Powertrain & Driveline
  note: Brakes
  note: Longitudinal Command Logic
  Acc : Inport
  Decel : Inport  Port=2
  VehFdbk : Inport  Port=3
  Brake System : Subsystem
  Brakes and Wheels : Subsystem  TreatAsAtomicUnit=on
      mask Display: image('vdbslibwhls.png');
  Bus Selector : BusSelector  OutputSignals=BdyFrm.FrntAxl.Lft.Vel.xdot,BdyFrm.FrntAxl.Rght.Vel.xdot,BdyFrm.RearAxl.Lft.Vel.xdot,BdyFrm.RearAxl.Rght.Vel.xdot
  Bus Selector1 : BusSelector  OutputSignals=BdyFrm.Forces.FrntAxl.Lft.Fz,BdyFrm.Forces.FrntAxl.Rght.Fz,BdyFrm.Forces.RearAxl.Lft.Fz,BdyFrm.Forces.RearAxl.Rght.Fz
  Bus Selector3 : BusSelector  OutputSignals=BdyFrm.FrntAxl.Steer.WhlAngFL,BdyFrm.FrntAxl.Steer.WhlAngFR,BdyFrm.RearAxl.Steer.WhlAngRL,BdyFrm.RearAxl.Steer.WhlAngRR  OutputAsBus=on
  Bus to Vector : BusToVector
  Constant : Constant  Value=-1
  Demux1 : Demux  Outputs=[2 2]
  Driveline : Subsystem  Variant=on  VariantControlMode=Label  VariantControl=Variant1  LabelModeActiveChoice=0
  Mux : Mux
  Mux1 : Mux
  Powertrain : Subsystem
  Suspension : autolibutils/Cont LPF  wc=10*pi*2  aMode=2
      settings: SourceProductBaseCode=PW,MT,AR,VE,VP
  Switch1 : Switch  Criteria=u2 > Threshold
  Switch2 : Switch  Criteria=u2 > Threshold
  Front Force : Outport  VectorParamsAs1DForOutWhenUnconnected=off
  Rear Force : Outport  Port=2  VectorParamsAs1DForOutWhenUnconnected=off
  wires:
  Brake System/1(Prs) -> Brakes and Wheels/2(BrkPrs)
  Switch2/1 -> Brake System/1(Decc)
  [Omega] -> Powertrain/3(Omega)
  [AxlPwr] -> Powertrain/2(AxlPwr)
  Brakes and Wheels/2(Omega) -> [Omega]
  Powertrain/1(AxlTrq) -> Driveline/1(TPowertrain)
  Switch1/1 -> Powertrain/1(Acc)
  Bus Selector1/4 -> Mux1/4  "<Fz>"
  Bus Selector1/3 -> Mux1/3  "<Fz>"
  Bus Selector1/2 -> Mux1/2  "<Fz>"
  Bus Selector1/1 -> Mux1/1  "<Fz>"
  Bus Selector/4 -> Mux/4  "<xdot>"
  Bus Selector/3 -> Mux/3  "<xdot>"
  Bus Selector/2 -> Mux/2  "<xdot>"
  Bus Selector/1 -> Mux/1  "<xdot>"
  Suspension/1 -> Brakes and Wheels/4(Fz)
  Mux1/1 -> Suspension/1
  Bus to Vector/1 -> Brakes and Wheels/5(delta)  "Steering"
  Bus Selector3/1 -> Bus to Vector/1
  Brakes and Wheels/3(Fx) -> Demux1/1
  Brakes and Wheels/1(AxlPwr) -> [AxlPwr]
  Driveline/1(TAxles) -> Brakes and Wheels/1(AxlTrq)
  Demux1/2 -> Rear Force/1
  Demux1/1 -> Front Force/1
  VehFdbk/1 -> Bus Selector/1, Bus Selector1/1, Bus Selector3/1
  Mux/1 -> Brakes and Wheels/3(Vx)  "WhlVel"
  Constant/1 -> Switch1/1, Switch2/3
  Acc/1 -> Switch1/3
  Decel/1 -> Switch2/1, Switch2/2, Switch1/2

== system vehicles/vehicle 1/Rate Transition1 ==
  Info : Inport
  Bus Selector2 : BusSelector  OutputSignals=InertFrm.Geom.Disp.X,InertFrm.Geom.Disp.Y,InertFrm.Cg.Ang.psi
  Derivative : Derivative
  Rate Transition1 : RateTransition  InitialCondition=X_o  OutPortSampleTime=0.01
  Rate Transition2 : RateTransition  InitialCondition=Y_o  OutPortSampleTime=0.01
  Rate Transition3 : RateTransition  OutPortSampleTime=0.01
  Scope3 : Scope
  X : Outport
  Y : Outport  Port=2
  Yaw : Outport  Port=3
  wires:
  Info/1 -> Bus Selector2/1
  Rate Transition3/1 -> Yaw/1
  Rate Transition2/1 -> Y/1
  Rate Transition1/1 -> X/1
  Bus Selector2/1 -> Rate Transition1/1  "<X>"
  Bus Selector2/3 -> Derivative/1, Rate Transition3/1  "<psi>"
  Bus Selector2/2 -> Rate Transition2/1  "<Y>"
  Derivative/1 -> Scope3/1

== system vehicles/vehicle 1/VelRefController1 ==
  angVel : Inport
  Abs : Abs
  Add : Sum  Inputs=+-
  Constant : Constant  Value=12
  Constant3 : Constant  Value=3
  Gain : Gain  Gain=80
  Relational Operator2 : RelationalOperator  OutDataTypeStr=boolean  RndMeth=Simplest
  Switch1 : Switch  Criteria=u2 > Threshold
  VelRef : Outport
  wires:
  angVel/1 -> Abs/1
  Gain/1 -> Add/2
  Abs/1 -> Gain/1
  Switch1/1 -> VelRef/1
  Constant/1 -> Add/1
  Relational Operator2/1 -> Switch1/2
  Constant3/1 -> Switch1/1, Relational Operator2/1
  Add/1 -> Switch1/3, Relational Operator2/2

== system vehicles/vehicle 1/Waypoints1 ==
  Constant3 : Constant  Value=xRef1  SampleTime=0.1
  Constant4 : Constant  Value=yRef1  SampleTime=0.1
  Matrix Concatenate : Concatenate  Mode=Multidimensional array  ConcatenateDimension=2
  WayPoints : Outport
  wires:
  Constant4/1 -> Matrix Concatenate/2
  Constant3/1 -> Matrix Concatenate/1
  Matrix Concatenate/1 -> WayPoints/1

== system vehicles/vehicle 10/Bus to Mux1 ==
  Info : Inport
  Bus Selector1 : BusSelector  OutputSignals=InertFrm.Cg.Disp.X,InertFrm.Cg.Disp.Y,InertFrm.Cg.Ang.psi
  Mux : Mux  Inputs=3
  Pose : Outport
  x : Outport  Port=2
  y : Outport  Port=3
  wires:
  Info/1 -> Bus Selector1/1
  Bus Selector1/2 -> Mux/2, y/1  "<Y>"
  Mux/1 -> Pose/1
  Bus Selector1/1 -> x/1, Mux/1  "<X>"
  Bus Selector1/3 -> Mux/3  "<psi>"

== system vehicles/vehicle 10/Concatenate1 ==
  delta : Inport
  Matrix Concatenate : Concatenate
  AnF : Outport  VectorParamsAs1DForOutWhenUnconnected=off
  wires:
  delta/1 -> Matrix Concatenate/1, Matrix Concatenate/2
  Matrix Concatenate/1 -> AnF/1

== system vehicles/vehicle 10/Lateral and Longitudinal Controller1 ==
  Waypoints : Inport
  Grade : Inport  Port=2
  Pose : Inport  Port=3
  VelRef : Inport  Port=4
  VelFdbk : Inport  Port=5
  xCar : Inport  Port=6
  yCar : Inport  Port=7
  Longitudinal Driver : autolibshared/Longitudinal Driver  extAccelOvr=off  extDecelOvr=off  extAccelHld=off  extDecelHld=off  extAccelZero=off  extDecelZero=off  cntrlType=PI  shftType=None  velUnits=m/s  gearOut=off  Kp=700  Ki=1  Kff=.1  Kg=0  VehVelVec=[0 100]  KffVec=[.1 .1]  KpVec=[10 10]  KiVec=[5 5]  KgVec=[0 0]  m=1500  Kpt=3000  tau=.1  L=2  aR=200  bR=2.5  cR=.5  g=9.81  vnom=9  Kaw=1  tauerr=.01  tauPt=2  GearInit=0  tShift=.1  pdlVec=[0.1 0.4 0.5 0.9]  upShftTbl=[-1 12.9375 26.4375 39.9375 51.18749999999999 62.4375 72.84375 83.25;-1 16.3125 29.8125 43.3125 54.5624 65.8125 76.78125 87.75;-1 19.6875 33.1875 46.68749999999999 57.9375 69.1875 80.71875 92.25;-1 33 52.5 77.25 100.5 138.75 161.875 185]  dwnShftTbl=[1 9.5625 23.0625 36.5625 47.8125 59.0625 68.90625 78.75;1 12.9375 26.4375 39.9375 51.18749999999999 62.4375 72.84375 83.25;1 16.3125 29.8125 43.3125 54.562499 65.8125 76.78125 87.75;1 19.6875 33.1875 46.68749999999999 57.9375 69.1875 80.71875 92.25]  tClutch=.5  tRev=.5  tPark=120  aMode=2  UpGearVec="[0  1  2  3  4  5  6  7]"  DownGearVec="[1  2  3  4  5  6  7  8]"
      settings: SourceProductBaseCode=PW,MT,VE,VP
  Pure Pursuit Controller : Subsystem
  Scope : Scope
  Scope1 : Scope
  Stop-system : Subsystem
  Terminator10 : Terminator
  angVel : Outport
  WheelSteeringAngle : Outport  Port=2
  AcelCmd : Outport  Port=3
  DecelCmd : Outport  Port=4
  wires:
  Stop-system/2(DecelCmd) -> DecelCmd/1, Scope1/1
  Stop-system/1(AcelCmd) -> AcelCmd/1, Scope/1
  yCar/1 -> Stop-system/4(yCar)
  xCar/1 -> Stop-system/2(xCar)
  Pure Pursuit Controller/2(AngularVelocity) -> angVel/1
  Longitudinal Driver/1 -> Terminator10/1
  Longitudinal Driver/2 -> Stop-system/1(acel)
  VelFdbk/1 -> Longitudinal Driver/2
  VelRef/1 -> Longitudinal Driver/1
  Longitudinal Driver/3 -> Stop-system/3(decel)
  Grade/1 -> Longitudinal Driver/3
  Pose/1 -> Pure Pursuit Controller/1(Pose)
  Waypoints/1 -> Pure Pursuit Controller/2(Waypoints)
  Pure Pursuit Controller/1(delta) -> WheelSteeringAngle/1
